simulink library "LopesDevelopmentLibrary"  (R2015b)
settings: Solver=ode45  StartTime=0.0  StopTime=10.0  RelTol=1e-3
values from neighbouring files (symbols this model uses):
  d2r = @(d) d*(pi/180)    [LopesDevelopmentLibrary_LoadParameters.m]
  ts = LopesParams.ts    [LopesDevelopmentLibrary_LoadParameters.m]
undefined symbols (not defined in the file or in its folder): anyParameterChanged, DiscIntNeverNeededParam, gcbh, LHF, LKF, LopesParams, macaddr, mxpcnetworkconfig, mxpcrtudprx, mxpcrtudptx, patientParametersChanged, port, PX, PZ, RHF, RKF, SelectorLOPESInSize, StrideTime_s, Time
undefined symbols (not defined in the file): LopesParamsSendDataArrayLen
libraries: LopesDevelopmentLibrary x288, simulink x98, dspmtrx3 x47, xpciplib x6, xpcnetworkbufferlib x5, dspsigops x4, dspstat3 x3, xpcethernetlib x2, visionstatistics x2, xpcseriallib x2, nmc x1, simulink_extras x1
(part 7 of 12)

== system LopesDevelopmentLibrary/Robot control blocks/ToLopes/GenerateString ==
  note: MaxForces is an array of maximum joint
      | torques and applies to SpringSpring
      | and BiasForceSpring separately.
  UpdateSpringPositions : Inport
  SpringPositions : Inport  Port=2
  SpringVelocities : Inport  Port=3
  SpringStiffnesses : Inport  Port=4
  BiasForces : Inport  Port=5
  MaxForces : Inport  Port=6
  EffectsShouldBeEnabled : Inport  Port=7
  ForceSendEnableEffects : Inport  Port=8
  TreadmillVelocity : Inport  Port=9
  CreateSpringspring : Inport  Port=10
  CreateBiasForceSpring : Inport  Port=11
  Enable : EnablePort
  Detect Change : simulink/Logic and Bit Operations/Detect Change  vinit=0  InputProcessing=Inherited  OutDataTypeStr=boolean
  Detect Change1 : simulink/Logic and Bit Operations/Detect Change  vinit=0  InputProcessing=Inherited  OutDataTypeStr=boolean
  Detect Increase : simulink/Logic and Bit Operations/Detect Increase  vinit=0.0  InputProcessing=Inherited  OutDataTypeStr=boolean
  ForceSendTreadmillVelocity : Constant  Value=false  OutDataTypeStr=boolean
      settings: OpenFcn=|
      | b = get_param(gcb,'value');
      | if (strcmp(b,'true')),
      |   set_param (gcb,'value','false');
      | else
      |   set_param(gcb,'value','true');
      | end;
  Or : Logic  Operator=OR  Inputs=1  AllPortsSameDT=off  OutDataTypeStr=boolean
  OrEnableEffects : Logic  Operator=OR  AllPortsSameDT=off  OutDataTypeStr=boolean
  OrTreadmill : Logic  Operator=OR  AllPortsSameDT=off  OutDataTypeStr=boolean
  ToLopes_GenerateString : S-Function  InitFcn=try, set_param(gcb,'FunctionName','ToLopes_GenerateString'), end  FunctionName=ToLopes_GenerateString  SFunctionModules=ToLopes_GenerateString_wrapper  SFunctionDeploymentMode=off  EnableBusSupport=off  mask(S-Function Builder){}
      mask help: Simulink:masks:SFunctionBuilder_MD
      mask init: same as LopesDevelopmentLibrary/Various/SLRTMessage/S-Function Builder
      settings: CopyFcn=set_param(gcbh,'LinkStatus','none')  PreSaveFcn=try, set_param(gcb,'FunctionName','ToLopes_GenerateString'), end  OpenFcn=sfunctionwizard(gcbh)
      mask Display: plot(val(:,1),val(:,2)),disp(sys), port_label('input',1,'UpdateSpringSpringPositions'), port_label('input',2,'SpringPositions'), port_label('input',3,'SpringVelocities'), port_label('input',4,'SpringStiffnesses'), port_label('input',5,'BiasForces'), port_label('input',6,'MaxForces'), port_label('input',7,'UpdateMaxForces'), port_label('input',8,'TreadmillVelocity'), port_label('input',9,'TreadmillVelocityChanged'), port_label('input',10,'CreateSpringSpring'), port_label('input',11,'CreateBiasForceSpring'), port_label('input',12,'EnableEffects'), port_label('output',1,'s'), port_label('output',2,'s_len')
  s : Outport
  s_len : Outport  Port=2
  wires:
  UpdateSpringPositions/1 -> ToLopes_GenerateString/1
  OrEnableEffects/1 -> ToLopes_GenerateString/12
  Detect Increase/1 -> OrEnableEffects/1
  EffectsShouldBeEnabled/1 -> Detect Increase/1
  ForceSendTreadmillVelocity/1 -> OrTreadmill/2
  OrTreadmill/1 -> ToLopes_GenerateString/9
  Detect Change1/1 -> OrTreadmill/1
  TreadmillVelocity/1 -> ToLopes_GenerateString/8, Detect Change1/1
  SpringVelocities/1 -> ToLopes_GenerateString/3
  Or/1 -> ToLopes_GenerateString/7
  Detect Change/1 -> Or/1
  MaxForces/1 -> ToLopes_GenerateString/6, Detect Change/1
  ForceSendEnableEffects/1 -> OrEnableEffects/2
  CreateSpringspring/1 -> ToLopes_GenerateString/10
  CreateBiasForceSpring/1 -> ToLopes_GenerateString/11
  SpringPositions/1 -> ToLopes_GenerateString/2
  SpringStiffnesses/1 -> ToLopes_GenerateString/4
  ToLopes_GenerateString/2 -> s_len/1
  ToLopes_GenerateString/1 -> s/1
  BiasForces/1 -> ToLopes_GenerateString/5

== system LopesDevelopmentLibrary/Robot control blocks/ToLopes/GenerateVelocities ==
  note: This block allows you to choose different sources for the
      | velocity component of the springspring. Normal behaviour
      | (when ForceVelocityMethod=-1) is that it will use the user-provided
      | velocity if that is an 8-element array, and it will
      | use numerical derivative of the position signal if it the velocity input
      | is a scalar (i.e., in order to use the numerical derivative, you just need to
      | give a scalar constant at the input).
  note: ForceVelocityMethod:
      | -1: Auto (use user-proved velocities if available; use numerical derivative otherwise)
      | 0: ERROR
      | 1: User velocities
      | 2. Numerical Derivatives
      | 3. Filtered numerical derivatives (tau=0.01 s)
      | 4. Zero velocity
  Positions : Inport
  Velocities : Inport  Port=2
  SignalWidth : Inport  Port=3
  ForceVelocityMethod : Inport  Port=4
  Demux : Demux
  MATLAB Function : MATLAB Function  TreatAsAtomicUnit=on
  Merge : Merge  Inputs=4
  UseNumericalDerivative : Subsystem  TreatAsAtomicUnit=on
  UseNumericalDerivativeFiltered : Subsystem  TreatAsAtomicUnit=on
  UseUserVelocity : Subsystem  TreatAsAtomicUnit=on
  UseZeros : Subsystem  TreatAsAtomicUnit=on
  v_out : Outport
  wires:
  Velocities/1 -> UseUserVelocity/1(Velocities_in)
  SignalWidth/1 -> MATLAB Function/1(signalWidth)
  Demux/1 -> UseUserVelocity/Enable
  Positions/1 -> UseNumericalDerivative/1(Positions), UseNumericalDerivativeFiltered/1(Positions)
  Demux/2 -> UseNumericalDerivative/Enable
  ForceVelocityMethod/1 -> MATLAB Function/2(forceType)
  MATLAB Function/1(ena) -> Demux/1
  Demux/4 -> UseZeros/Enable
  Demux/3 -> UseNumericalDerivativeFiltered/Enable
  UseNumericalDerivativeFiltered/1(Velocities) -> Merge/3
  UseZeros/1(Velocities) -> Merge/4
  UseNumericalDerivative/1(Velocities) -> Merge/2
  UseUserVelocity/1(Velocities) -> Merge/1
  Merge/1 -> v_out/1

== system LopesDevelopmentLibrary/Robot control blocks/ToLopes/ParseString ==
  s : Inport
  In2 : Inport  Port=2
  Enable : EnablePort
  ToLopes_ParseString : S-Function  InitFcn=try, set_param(gcb,'FunctionName','ToLopes_ParseString'), end  FunctionName=ToLopes_ParseString  SFunctionModules=ToLopes_ParseString_wrapper  SFunctionDeploymentMode=off  EnableBusSupport=off  mask(S-Function Builder){}
      mask help: Simulink:masks:SFunctionBuilder_MD
      mask init: same as LopesDevelopmentLibrary/Various/SLRTMessage/S-Function Builder
      settings: CopyFcn=set_param(gcbh,'LinkStatus','none')  PreSaveFcn=try, set_param(gcb,'FunctionName','ToLopes_ParseString'), end  OpenFcn=sfunctionwizard(gcbh)
      mask Display: plot(val(:,1),val(:,2)),disp(sys), port_label('input',1,'s'), port_label('input',2,'s_len'), port_label('output',1,'ErrorValue'), port_label('output',2,'SpringSpringDidntExist'), port_label('output',3,'BiasForceSpringDidntExist')
  Error : Outport
  SpringSpringDidntExist : Outport  Port=2
  BiasForceSpringDidntExist : Outport  Port=3
  wires:
  ToLopes_ParseString/3 -> BiasForceSpringDidntExist/1
  ToLopes_ParseString/2 -> SpringSpringDidntExist/1
  ToLopes_ParseString/1 -> Error/1
  s/1 -> ToLopes_ParseString/1
  In2/1 -> ToLopes_ParseString/2

== system LopesDevelopmentLibrary/Robot control blocks/ToLopes/SwitchVelocitiesOnly ==
  note: This block contains the logic for
      | using 'velocity only' control.
      | You should ONLY use it if
      | you have analytical derivatives of your
      | positions. If you have analytical second derivatives
      | as well, it will be more accurate
      | (use the block Various|BetterSpringVelocities)
      |
      | NOTE: UseAnalyticalVelocityOnly is more accurate (i.e., better),
      | but only usable if you have correct derivatives.
  note: The UseAnalyticalVelocityOnly block does not work properly
      | and (thus) should not be used until it's fixed. Please use the positions-and-velocity
      | mode.
      |
      | (the reason this doesn't work: I'm comparing the DesiredSpringPos with the ModelPosIn,
      | but I should compare it to the ActualSpringPos. I don't read that from the LLC yet, and adding
      | this requires some testing. So it is not a 1-minute fix.) - GvO, 151215
  UseAnalVelOnly : Inport
  ModelPosIn : Inport  Port=2
  DesSprPos : Inport  Port=3
  DesSprVel : Inport  Port=4
  Logical Operator : Logic  Operator=NOT  AllPortsSameDT=off  OutDataTypeStr=boolean
  Merge : Merge
  Merge1 : Merge
  Merge2 : Merge
  UseAnalyticalVelocityOnly : Subsystem
  UsePositionsAndVelocities : Subsystem
  UpdateSpringPos : Outport
  SpringPositions : Outport  Port=2
  SpringVelocities : Outport  Port=3
  wires:
  Logical Operator/1 -> UsePositionsAndVelocities/Enable
  UseAnalVelOnly/1 -> UseAnalyticalVelocityOnly/Enable, Logical Operator/1
  DesSprVel/1 -> UsePositionsAndVelocities/2(DesSprVel), UseAnalyticalVelocityOnly/3(DesSprVel)
  DesSprPos/1 -> UsePositionsAndVelocities/1(DesSprPos), UseAnalyticalVelocityOnly/2(DesSprPos)
  ModelPosIn/1 -> UseAnalyticalVelocityOnly/1(ModelPosIn)
  UsePositionsAndVelocities/3(SpringVelocities) -> Merge2/2
  UseAnalyticalVelocityOnly/3(SpringVelocities) -> Merge2/1
  UsePositionsAndVelocities/2(SpringPositions) -> Merge1/2
  UseAnalyticalVelocityOnly/2(SpringPositions) -> Merge1/1
  UsePositionsAndVelocities/1(UpdateSpringPos) -> Merge/2
  UseAnalyticalVelocityOnly/1(UpdateSpringPos) -> Merge/1
  Merge1/1 -> SpringPositions/1
  Merge2/1 -> SpringVelocities/1
  Merge/1 -> UpdateSpringPos/1

== system LopesDevelopmentLibrary/Robot control blocks/ToLopes/~Debug ==

== system LopesDevelopmentLibrary/Robot control blocks/ToLopes/~EnableLogic ==

== system LopesDevelopmentLibrary/Various/GenerateSyncPulseFromPhase/DetectPhaseSignalReset ==
  note: This block detects the event of phase reset (i.e., when it
      | goes from (approximately) 100 to (approximately) 0.
      | It does this by checking whether there is a decrease of at
      | least 50% within one sample time.
  Phase : Inport
  Compare To Constant : simulink/Logic and Bit Operations/Compare To Constant  relop=<  const=-50  OutDataTypeStr=boolean
  Subtract : Sum  Inputs=+-
  Unit Delay : UnitDelay  SampleTime=-1
  PhaseReset : Outport
  wires:
  Phase/1 -> Subtract/1, Unit Delay/1
  Compare To Constant/1 -> PhaseReset/1
  Unit Delay/1 -> Subtract/2
  Subtract/1 -> Compare To Constant/1

== system LopesDevelopmentLibrary/Various/GenerateSyncPulseFromPhase/GenerateRandomValue ==
  note: Generate a uniform random number between Minimum and Maximum each
      | time Trigger rises.
  Maximum : Inport
  Minimum : Inport  Port=2
  Trigger : TriggerPort  PortDimensions=1
  Add : Sum
  Product : Product  RndMeth=Zero
  Subtract : Sum  Inputs=+-
  Uniform Random Number : UniformRandomNumber  Minimum=0  Seed=66
  Out : Outport  InitialOutput=0
  wires:
  Maximum/1 -> Subtract/1
  Uniform Random Number/1 -> Product/1
  Product/1 -> Add/1
  Subtract/1 -> Product/2
  Add/1 -> Out/1
  Minimum/1 -> Add/2, Subtract/2

== system LopesDevelopmentLibrary/BlocksForInternalUse/GaitGeneration/CalculateCartesianPositions/ConvertFromAnkleAnglesToFootAngles ==
  note: Input for s-function,
      | jointAngles:
      | PelvisPosX
      | PelvixPosY
      | PelvisPosZ
      | PelvisAxialAngle
      | PelvisFrontalAngle
      | LHA
      | LHF
      | LHEndorotatoin
      | LKF
      | LAEndorotation
      | LAP
      | LAInversion
      | RHA
      | RHF
      | RHEnorotation
      | RKF
      | RAEndorotation
      | RAP
      | RAInversion
  note: The S-function uses absolute angles for the ankle angle,
      | and I use relative angles (relative to the lower leg).
      | This part converts it. It would be better to use
      | the same thing in both software parts however.
      | (but as long as we don't actuate/measure the ankle
      | angle, it doesn't matter at all.
  In : Inport
  Demux1 : Demux  Outputs=11
  Mux1 : Mux  Inputs=19
  Zero{,1..7} (8 alike) : Constant  Value=0
  Out : Outport
  wires:
  Zero7/1 -> Mux1/19  "RAI"
  Zero6/1 -> Mux1/18  "RAP"
  Zero5/1 -> Mux1/17  "RAE"
  Demux1/8 -> Mux1/16  "RKF"
  Zero4/1 -> Mux1/15  "RHE"
  Demux1/7 -> Mux1/14  "RHF"
  Demux1/6 -> Mux1/13  "RHA"
  Zero3/1 -> Mux1/12  "LAI"
  Zero2/1 -> Mux1/11  "LAP"
  Zero1/1 -> Mux1/10  "LAE"
  Demux1/5 -> Mux1/9  "LKF"
  Zero/1 -> Mux1/8  "LHE"
  Demux1/4 -> Mux1/7  "LHF"
  Demux1/3 -> Mux1/6  "LHA"
  Demux1/11 -> Mux1/5  "POB"
  Demux1/10 -> Mux1/4  "PAX"
  Demux1/9 -> Mux1/2  "PY"
  Demux1/2 -> Mux1/3  "PZ"
  Demux1/1 -> Mux1/1  "PX"
  In/1 -> Demux1/1
  Mux1/1 -> Out/1

== system LopesDevelopmentLibrary/BlocksForInternalUse/GaitGeneration/CalculateCartesianPositions/ExtractPatientParameters ==
  Parameters : Inport
  Bus Selector : BusSelector  OutputSignals=Patient.Mass_kg,Patient.BodyLength_m,Patient.PelvisWidth_m,Patient.PelvisHeight_m,Patient.UpperLegLength_m,Patient.LowerLegLength_m,Patient.FootLength_m,Patient.FootHeight_m,patientParametersChanged
  Data Type Conversion : DataTypeConversion  OutDataTypeStr=double
  Mux : Mux  Inputs=12
  PatientDimensions : Outport
  DimensionsChanged : Outport  Port=2
  wires:
  Data Type Conversion/1 -> DimensionsChanged/1
  Bus Selector/8 -> Mux/11, Mux/12  "<FootHeight_m>"
  Bus Selector/2 -> Mux/2  "<BodyLength_m>"
  Bus Selector/5 -> Mux/6, Mux/5  "<UpperLegLength_m>"
  Bus Selector/3 -> Mux/3  "<PelvisWidth_m>"
  Bus Selector/1 -> Mux/1  "<Mass_kg>"
  Bus Selector/7 -> Mux/9, Mux/10  "<FootLength_m>"
  Bus Selector/9 -> Data Type Conversion/1  "<patientParametersChanged>"
  Mux/1 -> PatientDimensions/1
  Bus Selector/6 -> Mux/7, Mux/8  "<LowerLegLength_m>"
  Parameters/1 -> Bus Selector/1
  Bus Selector/4 -> Mux/4  "<PelvisHeight_m>"

== system LopesDevelopmentLibrary/BlocksForInternalUse/GaitGeneration/CalculateCartesianPositions/OmitAnklesAndToes ==
  In : Inport
  Demux1 : Demux  Outputs=11
  Mux1 : Mux  Inputs=7
  Terminator{,1..3} (4 alike) : Terminator
  Out : Outport
  wires:
  Mux1/1 -> Out/1
  Demux1/10 -> Terminator2/1  "RightHeel"
  Demux1/11 -> Terminator3/1  "RightToe"
  Demux1/6 -> Terminator1/1  "LeftToe"
  Demux1/5 -> Terminator/1  "LeftHeel"
  Demux1/7 -> Mux1/5  "RightHip"
  Demux1/9 -> Mux1/7  "RightAnkle"
  Demux1/1 -> Mux1/1  "Pelvis"
  Demux1/2 -> Mux1/2  "LeftHip"
  Demux1/4 -> Mux1/4  "LeftAnkle"
  Demux1/8 -> Mux1/6  "RightKnee"
  In/1 -> Demux1/1
  Demux1/3 -> Mux1/3  "LeftKnee"

== system LopesDevelopmentLibrary/BlocksForInternalUse/GaitGeneration/CalculateReferenceGait/ActuatedDOFs ==

== system LopesDevelopmentLibrary/BlocksForInternalUse/GaitGeneration/CalculateReferenceGait/CalculateAbductionLeft ==
  note: This version of the CalculateAbduction calculates
      | the derivatives analytically. At the end of the script there is a (commented)
      | Matlab script that calculates the derivatives using the symbolic toolbox. It shows analytically that
      | the velocity is calculated correctly, and the acceleration is too complex to solve for.
      | For the acceleration, I put in random numbers as input and compared the result of my own (optimized) equation
      | and the equation found by Matla Symbolic toolbox. They are equal, so that proves that my equations are all okay.
  note: This block calculates the abduction angle for one leg, given the actual pelvis position and the desired ankle position.
      | It does not take into account rotations of the pelvis, but the deviations from that are so small that that is not a problem.
  Parameters : Inport
  PelvisTZ : Inport  Port=2
  AnkleTZ : Inport  Port=3
  xHF : Inport  Port=4
  xKF : Inport  Port=5
  Bus Selector : BusSelector  OutputSignals=Patient.PelvisWidth_m,Patient.UpperLegLength_m,Patient.LowerLegLength_m
  Demux{,1..3} (4 alike) : Demux  Outputs=3
  MATLAB Function : MATLAB Function  TreatAsAtomicUnit=on
  Signal Conversion : SignalConversion
  isRight : Constant  Value=isRight
  Abduction : Outport
  dAbduction_dx : Outport  Port=2
  d2Abduction_dx2 : Outport  Port=3
  wires:
  isRight/1 -> MATLAB Function/1(isRight)
  PelvisTZ/1 -> Demux/1
  AnkleTZ/1 -> Demux1/1
  xHF/1 -> Demux2/1
  xKF/1 -> Demux3/1
  Parameters/1 -> Bus Selector/1
  Bus Selector/1 -> MATLAB Function/14(w_pelvis)  "<PelvisWidth_m>"
  Bus Selector/2 -> MATLAB Function/15(l_upper)  "<UpperLegLength_m>"
  Bus Selector/3 -> MATLAB Function/16(l_lower)  "<LowerLegLength_m>"
  MATLAB Function/1(Abduction) -> Signal Conversion/1
  MATLAB Function/2(dAbductiondx) -> dAbduction_dx/1
  MATLAB Function/3(ddAbductiondx) -> d2Abduction_dx2/1
  Signal Conversion/1 -> Abduction/1
  Demux/2 -> MATLAB Function/3(dPelvisTZdx)
  Demux/3 -> MATLAB Function/4(ddPelvisTZdx)
  Demux/1 -> MATLAB Function/2(PelvisTZ)
  Demux1/2 -> MATLAB Function/6(dAnkleTZdx)
  Demux1/1 -> MATLAB Function/5(AnkleTZ)
  Demux1/3 -> MATLAB Function/7(ddAnkleTZdx)
  Demux2/2 -> MATLAB Function/9(dxHFdx)
  Demux2/3 -> MATLAB Function/10(ddxHFdx)
  Demux2/1 -> MATLAB Function/8(xHF)
  Demux3/3 -> MATLAB Function/13(ddxKFdx)
  Demux3/1 -> MATLAB Function/11(xKF)
  Demux3/2 -> MATLAB Function/12(dxKFdx)

== system LopesDevelopmentLibrary/BlocksForInternalUse/GaitGeneration/CalculateReferenceGait/CalculateAbductionRight ==
  note: This block calculates the abduction angle for one leg, given the actual pelvis position and the desired ankle position.
      | It does not take into account rotations of the pelvis, but the deviations from that are so small that that is not a problem.
  note: This version of the CalculateAbduction calculates
      | the derivatives analytically. At the end of the script there is a (commented)
      | Matlab script that calculates the derivatives using the symbolic toolbox. It shows analytically that
      | the velocity is calculated correctly, and the acceleration is too complex to solve for.
      | For the acceleration, I put in random numbers as input and compared the result of my own (optimized) equation
      | and the equation found by Matla Symbolic toolbox. They are equal, so that proves that my equations are all okay.
  Parameters : Inport
  PelvisTZ : Inport  Port=2
  AnkleTZ : Inport  Port=3
  xHF : Inport  Port=4
  xKF : Inport  Port=5
  Bus Selector : BusSelector  OutputSignals=Patient.PelvisWidth_m,Patient.UpperLegLength_m,Patient.LowerLegLength_m
  Demux{,1..3} (4 alike) : Demux  Outputs=3
  MATLAB Function : MATLAB Function  TreatAsAtomicUnit=on
  Signal Conversion : SignalConversion
  isRight : Constant  Value=isRight
  Abduction : Outport
  dAbduction_dx : Outport  Port=2
  d2Abduction_dx2 : Outport  Port=3
  wires:
  Demux3/2 -> MATLAB Function/12(dxKFdx)
  Demux3/1 -> MATLAB Function/11(xKF)
  Demux3/3 -> MATLAB Function/13(ddxKFdx)
  Demux2/1 -> MATLAB Function/8(xHF)
  Demux2/3 -> MATLAB Function/10(ddxHFdx)
  Demux2/2 -> MATLAB Function/9(dxHFdx)
  Demux1/3 -> MATLAB Function/7(ddAnkleTZdx)
  Demux1/1 -> MATLAB Function/5(AnkleTZ)
  Demux1/2 -> MATLAB Function/6(dAnkleTZdx)
  Demux/1 -> MATLAB Function/2(PelvisTZ)
  Demux/3 -> MATLAB Function/4(ddPelvisTZdx)
  Demux/2 -> MATLAB Function/3(dPelvisTZdx)
  Signal Conversion/1 -> Abduction/1
  MATLAB Function/3(ddAbductiondx) -> d2Abduction_dx2/1
  MATLAB Function/2(dAbductiondx) -> dAbduction_dx/1
  MATLAB Function/1(Abduction) -> Signal Conversion/1
  Bus Selector/3 -> MATLAB Function/16(l_lower)  "<LowerLegLength_m>"
  Bus Selector/2 -> MATLAB Function/15(l_upper)  "<UpperLegLength_m>"
  Bus Selector/1 -> MATLAB Function/14(w_pelvis)  "<PelvisWidth_m>"
  Parameters/1 -> Bus Selector/1
  xKF/1 -> Demux3/1
  xHF/1 -> Demux2/1
  AnkleTZ/1 -> Demux1/1
  PelvisTZ/1 -> Demux/1
  isRight/1 -> MATLAB Function/1(isRight)

== system LopesDevelopmentLibrary/BlocksForInternalUse/GaitGeneration/CalculateReferenceGait/FirstDerivativeWrtTime ==
  dydx : Inport
  dtdx : Inport  Port=2
  Divide : Product  Inputs=*/
  dydt : Outport
  wires:
  Divide/1 -> dydt/1
  dydx/1 -> Divide/1
  dtdx/1 -> Divide/2

== system LopesDevelopmentLibrary/BlocksForInternalUse/GaitGeneration/CalculateReferenceGait/SecondDerivativeWrtTime ==
  ddydx : Inport
  dtdx : Inport  Port=2
  Divide1 : Product  Inputs=*/
  Math Function : Math  Operator=square  SaturateOnIntegerOverflow=on
  ddydt : Outport
  wires:
  dtdx/1 -> Math Function/1
  Math Function/1 -> Divide1/2
  ddydx/1 -> Divide1/1
  Divide1/1 -> ddydt/1

== system LopesDevelopmentLibrary/BlocksForInternalUse/GaitGeneration/CalculateReferenceGait/Unactuated DOFS ==

== system LopesDevelopmentLibrary/BlocksForInternalUse/GaitGenerationStartStop/ExtraKeyPoints /LeftHipFlexion ==
  parameters : Inport
  SetVelocity : Inport  Port=2
  Bus Creator4 : BusCreator  Inputs=2
  Bus Selector : BusSelector  OutputSignals=General.WalkingVelocity_m_s,Patient.BodyLength_m
  RegressionData : Constant  Value=LopesParams.GaitDataStartLeft.LHF
  RegressionData2KeyEvents : LopesDevelopmentLibrary/BlocksForInternalUse/GaitGeneration/RegressionData2KeyEvents
  Switch : Switch  Criteria=u2 > Threshold
  KeyEvents : Outport
  wires:
  RegressionData2KeyEvents/1 -> KeyEvents/1
  parameters/1 -> Bus Selector/1
  RegressionData/1 -> RegressionData2KeyEvents/1
  Bus Creator4/1 -> RegressionData2KeyEvents/2
  Bus Selector/2 -> Bus Creator4/2  "<BodyLength_m>"
  Bus Selector/1 -> Switch/3  "<WalkingVelocity_m_s>"
  SetVelocity/1 -> Switch/2, Switch/1
  Switch/1 -> Bus Creator4/1  "WalkingVelocity_m_s"

== system LopesDevelopmentLibrary/BlocksForInternalUse/GaitGenerationStartStop/ExtraKeyPoints /LeftKneeFlexion ==
  parameters : Inport
  SetVelocity : Inport  Port=2
  Bus Creator4 : BusCreator  Inputs=2
  Bus Selector : BusSelector  OutputSignals=General.WalkingVelocity_m_s,Patient.BodyLength_m
  RegressionData : Constant  Value=LopesParams.GaitDataStartLeft.LKF
  RegressionData2KeyEvents : LopesDevelopmentLibrary/BlocksForInternalUse/GaitGeneration/RegressionData2KeyEvents
  Switch : Switch  Criteria=u2 > Threshold
  KeyEvents : Outport
  wires:
  RegressionData2KeyEvents/1 -> KeyEvents/1
  RegressionData/1 -> RegressionData2KeyEvents/1
  parameters/1 -> Bus Selector/1
  Bus Creator4/1 -> RegressionData2KeyEvents/2
  Bus Selector/2 -> Bus Creator4/2  "<BodyLength_m>"
  Bus Selector/1 -> Switch/3  "<WalkingVelocity_m_s>"
  SetVelocity/1 -> Switch/2, Switch/1
  Switch/1 -> Bus Creator4/1  "WalkingVelocity_m_s"

== system LopesDevelopmentLibrary/BlocksForInternalUse/GaitGenerationStartStop/ExtraKeyPoints /PelvisTPX ==
  parameters : Inport
  SetVelocity : Inport  Port=2
  Bus Creator4 : BusCreator  Inputs=2
  Bus Selector : BusSelector  OutputSignals=General.WalkingVelocity_m_s,Patient.BodyLength_m
  RegressionData : Constant  Value=LopesParams.GaitDataStartLeft.PX
  RegressionData2KeyEvents : LopesDevelopmentLibrary/BlocksForInternalUse/GaitGeneration/RegressionData2KeyEvents
  Switch : Switch  Criteria=u2 > Threshold
  KeyEvents : Outport
  wires:
  Switch/1 -> Bus Creator4/1  "WalkingVelocity_m_s"
  SetVelocity/1 -> Switch/1, Switch/2
  Bus Selector/1 -> Switch/3  "<WalkingVelocity_m_s>"
  Bus Selector/2 -> Bus Creator4/2  "<BodyLength_m>"
  Bus Creator4/1 -> RegressionData2KeyEvents/2
  RegressionData/1 -> RegressionData2KeyEvents/1
  parameters/1 -> Bus Selector/1
  RegressionData2KeyEvents/1 -> KeyEvents/1

== system LopesDevelopmentLibrary/BlocksForInternalUse/GaitGenerationStartStop/ExtraKeyPoints /PelvisTPZ ==
  parameters : Inport
  SetVelocity : Inport  Port=2
  Bus Creator4 : BusCreator  Inputs=2
  Bus Selector : BusSelector  OutputSignals=General.WalkingVelocity_m_s,Patient.BodyLength_m
  RegressionData : Constant  Value=LopesParams.GaitDataStartLeft.PZ
  RegressionData2KeyEvents : LopesDevelopmentLibrary/BlocksForInternalUse/GaitGeneration/RegressionData2KeyEvents
  Switch : Switch  Criteria=u2 > Threshold
  KeyEvents : Outport
  wires:
  Switch/1 -> Bus Creator4/1  "WalkingVelocity_m_s"
  SetVelocity/1 -> Switch/1, Switch/2
  Bus Selector/1 -> Switch/3  "<WalkingVelocity_m_s>"
  Bus Selector/2 -> Bus Creator4/2  "<BodyLength_m>"
  Bus Creator4/1 -> RegressionData2KeyEvents/2
  RegressionData/1 -> RegressionData2KeyEvents/1
  parameters/1 -> Bus Selector/1
  RegressionData2KeyEvents/1 -> KeyEvents/1

== system LopesDevelopmentLibrary/BlocksForInternalUse/GaitGenerationStartStop/ExtraKeyPoints /RightHipFlexion ==
  parameters : Inport
  SetVelocity : Inport  Port=2
  Bus Creator4 : BusCreator  Inputs=2
  Bus Selector : BusSelector  OutputSignals=General.WalkingVelocity_m_s,Patient.BodyLength_m
  RegressionData : Constant  Value=LopesParams.GaitDataStartLeft.RHF
  RegressionData2KeyEvents : LopesDevelopmentLibrary/BlocksForInternalUse/GaitGeneration/RegressionData2KeyEvents
  Switch : Switch  Criteria=u2 > Threshold
  KeyEvents : Outport
  wires:
  RegressionData/1 -> RegressionData2KeyEvents/1
  RegressionData2KeyEvents/1 -> KeyEvents/1
  parameters/1 -> Bus Selector/1
  Bus Creator4/1 -> RegressionData2KeyEvents/2
  Bus Selector/2 -> Bus Creator4/2  "<BodyLength_m>"
  Bus Selector/1 -> Switch/3  "<WalkingVelocity_m_s>"
  SetVelocity/1 -> Switch/2, Switch/1
  Switch/1 -> Bus Creator4/1  "WalkingVelocity_m_s"

== system LopesDevelopmentLibrary/BlocksForInternalUse/GaitGenerationStartStop/ExtraKeyPoints /RightKneeFlexion ==
  parameters : Inport
  SetVelocity : Inport  Port=2
  Bus Creator4 : BusCreator  Inputs=2
  Bus Selector : BusSelector  OutputSignals=General.WalkingVelocity_m_s,Patient.BodyLength_m
  RegressionData : Constant  Value=LopesParams.GaitDataStartLeft.RKF
  RegressionData2KeyEvents : LopesDevelopmentLibrary/BlocksForInternalUse/GaitGeneration/RegressionData2KeyEvents
  Switch : Switch  Criteria=u2 > Threshold
  KeyEvents : Outport
  wires:
  RegressionData2KeyEvents/1 -> KeyEvents/1
  RegressionData/1 -> RegressionData2KeyEvents/1
  parameters/1 -> Bus Selector/1
  Bus Creator4/1 -> RegressionData2KeyEvents/2
  Bus Selector/2 -> Bus Creator4/2  "<BodyLength_m>"
  Bus Selector/1 -> Switch/3  "<WalkingVelocity_m_s>"
  SetVelocity/1 -> Switch/2, Switch/1
  Switch/1 -> Bus Creator4/1  "WalkingVelocity_m_s"

== system LopesDevelopmentLibrary/BlocksForInternalUse/GaitGenerationStartStop/ExtraKeyPoints /TimeCalculation ==
  StrideTime : Inport
  Bus Creator7 : BusCreator  Inputs=2
  Constant : Constant  Value=[0,0,1; 100,1,1]
  Gain : Gain  Gain=0.01
  Mux : Mux  Inputs=2
  Overwrite Values : dspmtrx3/Overwrite Values  OverWriteDiag=Submatrix  valFrom2ndIP=Second input port  ConstValue=0  RowSpan=One row  RowStartMode=Index  RowStartIndex=2  RowEndMode=Last  RowEndIndex=1  ColSpan=One column  ColStartMode=Index  ColStartIndex=2  ColEndMode=Last  ColEndIndex=1  DiagSpan=Range of elements  DiagStartMode=Index  DiagStartIndex=2  DiagEndMode=Index  DiagEndIndex=4
  Overwrite Values1 : dspmtrx3/Overwrite Values  OverWriteDiag=Submatrix  valFrom2ndIP=Second input port  ConstValue=0  RowSpan=All rows  RowStartMode=Index  RowStartIndex=2  RowEndMode=Last  RowEndIndex=1  ColSpan=One column  ColStartMode=Last  ColStartIndex=2  ColEndMode=Last  ColEndIndex=1  DiagSpan=Range of elements  DiagStartMode=Index  DiagStartIndex=2  DiagEndMode=Index  DiagEndIndex=4
  Time : LopesDevelopmentLibrary/BlocksForInternalUse/GaitGeneration/keyEvents2breakscoefs3  SystemSampleTime=-1
  BreaksCoefsTime : Outport
  wires:
  StrideTime/1 -> Overwrite Values/2, Gain/1
  Overwrite Values1/1 -> Time/1
  Constant/1 -> Overwrite Values/1
  Overwrite Values/1 -> Overwrite Values1/1
  Mux/1 -> Overwrite Values1/2
  Gain/1 -> Mux/1, Mux/2  "slope"
  Time/2 -> Bus Creator7/2
  Time/1 -> Bus Creator7/1
  Bus Creator7/1 -> BreaksCoefsTime/1  "Time"

== system LopesDevelopmentLibrary/BlocksForInternalUse/LLC Communication/LLC Network Configuration/Variant Network Init ==
  note: 1) Only subsystems can be added as variant choices at this level
      | 2) Blocks cannot be connected at this level as connectivity is
      | automatically determined at simulation, based on the active variant
  note: I did not remove the inputs/outputs because that makes Matlab fail...
  Dummy_in : Inport
  Init_NonRT_UDP : Subsystem  VariantControl=LopesVariant_Non_RT
  Init_RT_2012b : Subsystem  VariantControl=LopesVariant_RT_2012b
  Init_RT_2014b : Subsystem  VariantControl=LopesVariant_RT_2014b
  Init_RT_2015b : Subsystem  VariantControl=LopesVariant_RT_2015b
  Dummy_out : Outport

== system LopesDevelopmentLibrary/BlocksForInternalUse/LLC Communication/LLCReceiveUDP/Debug ==

== system LopesDevelopmentLibrary/BlocksForInternalUse/LLC Communication/LLCReceiveUDP/UDPReceiveVariantChannel ==
  note: 1) Add Subsystem or Model blocks as valid variant choices.
      | 2) You cannot connect blocks at this level. At simulation, connectivity is automatically
      | determined, based on the active variant and port name matching.
  Dummy_in : Inport
  Receive_Non_RT : Subsystem  VariantControl=LopesVariant_Non_RT
  Receive_RT_2015b : Subsystem  VariantControl=LopesVariant_RT_2015b
  Receive_RT_R2012b : Subsystem  VariantControl=LopesVariant_RT_2012b
  Receive_RT_R2014b : Subsystem  VariantControl=LopesVariant_RT_2014b
  RecvData : Outport
  RecvLen : Outport  Port=2

== system LopesDevelopmentLibrary/BlocksForInternalUse/LLC Communication/LLCSendUDP/Debug ==

== system LopesDevelopmentLibrary/BlocksForInternalUse/LLC Communication/LLCSendUDP/UDPSendVariant ==
  Data : Inport
  Len : Inport  Port=2
  Enable : EnablePort
  Terminator : Terminator
  UDPSendVariantChannel : Subsystem  Variant=on
  wires:
  Data/1 -> UDPSendVariantChannel/1(SendData)
  Len/1 -> UDPSendVariantChannel/2(SendLen)
  UDPSendVariantChannel/1(Dummy_out) -> Terminator/1

== system LopesDevelopmentLibrary/BlocksForInternalUse/LLC Communication/UDP_Blocks/Network Configuration_RT_2012b  ==
  "ARP Init " : S-Function  Priority=0  FunctionName=xpcdebugarpinit  Parameters=Stats, Interface, IpAddress, SubnetMask, Gateway, EthernetId, Flags, BlockId, Retry, Timeout, Expiration, StaticAddressListIp, StaticAddressListMac, DiscoveryList, MulticastList, SampleTime  SFunctionDeploymentMode=off  EnableBusSupport=off  mask(arpinit){Interface=0, IpAddress=IpAddress, SubnetMask=SubnetMask, Gateway=Gateway, EthernetId=1, BlockId=0, SampleTime=-1, Flags=hex2dec('00000697'), Stats=off, Retry=5, Timeout=20, Expiration=20*60, StaticAddressListIp=[], StaticAddressListMac=[], DiscoveryList=[], MulticastList=[]}
      mask prompts: IpAddress "IP Address"; SubnetMask "Subnet Mask"; EthernetId "Ethernet ID"; BlockId "Block ID"; SampleTime "Sample Time"; Stats "Statistics Port"; StaticAddressListIp "[Static IP]"; StaticAddressListMac "[Static MAC]"; DiscoveryList "[Discovery IP]"; MulticastList "[Multicast IP]"
      mask help: ARP Init
      mask init:
      | xpclinklib('xpciplib');
      mask Help: web('arpdebug.htm',  '-helpbrowser');
      mask Display: disp('ARP Init');
  "Buffer Mngmt " : S-Function  Priority=-1  FunctionName=xpcnb  Parameters=pool_sizes, SampleTime, ShowTune  SFunctionDeploymentMode=off  EnableBusSupport=off  mask(xpcnbinit){SampleTime=-1, PoolSizes=[100 10 10 200], ShowTune=off}
      mask prompts: SampleTime "Sample time:"; PoolSizes "Buffer pool sizes (256, 512, 1024, 2048):"; ShowTune "Display tuning information"
      mask help: Network Buffer Initialization
      mask init:
      | [MaskDisplay, pool_sizes] = mxpcnbinit(2, PoolSizes);
      | 
      | set_param(gcb, 'MaskDisplay', MaskDisplay);
      mask Help: eval('xpcdoc(''NB_Init'')');
      mask Display: disp('Network Buffer\nManagement');
  "Ethernet Init " : S-Function  Priority=-1  FunctionName=xpcetherinit  Parameters="ID, Driver, Bus, Slot, VendorID, DeviceID, AddressSource, mac, TxSA, RxPromiscuous, RxBad, RxShort, MaxMTU, TxThreshold, TxBuffers, RxBuffers, ShowTune, numMulti, multicast,   NumRxBlks, SampleTime"  SFunctionDeploymentMode=off  EnableBusSupport=off  mask(xpcetherinit){ID=1, Driver=EthDrv, Bus=PciBus, Slot=PciSlot, SampleTime=-1, AddressSource=EEPROM, MAC=macaddr('00:00:00:00:00:00'), TxSA=off, RxPromiscuous=off, Multicast={}, RxBad=off, RxShort=off, MaxMTU=1518, TxThreshold=224, TxBuffers=128, RxBuffers=64, ShowTune=off, NumRxBlks=1}
      mask prompts: ID "Device ID:"; Bus "PCI bus:"; Slot "PCI slot:"; SampleTime "Sample time:"; AddressSource "Address source:"; TxSA "Tx source address from model"; RxPromiscuous "Rx promiscuous"; Multicast "Multicast address list:"; RxBad "Rx bad frames"; RxShort "Rx short frames"; MaxMTU "Max MTU:"; TxThreshold "Tx threshold:"; TxBuffers "Tx buffers:"; RxBuffers "Rx buffers:"; ShowTune "Display tuning information"; NumRxBlks "num rx blocks"
      mask help: Ethernet Initialization
      mask init:
      | VendorID = -1;
      | DeviceID = -1;
      | 
      | [MaskDisplay, VendorID, DeviceID, mac, numMulti, multicast] = mxpcetherinit(2, ID, Driver, Bus, Slot, MAC, Multicast);
      | 
      | set_param(gcb, 'MaskDisplay', MaskDisplay);
      mask Help: eval('xpcdoc(''Ether_Init'')');
      mask TypeOptions ID: 1 | 2 | 3 | 4 | 5 | 6 | 7 | 8
      mask TypeOptions AddressSource: EEPROM | Specify
      mask Callback AddressSource:
      | enables = get_param(gcb, 'MaskVisibilities');
      | if strcmp('Specify', get_param(gcb, 'AddressSource'))
      |     enables{strmatch('MAC',fieldnames(get_param(gcb,'DialogParameters')))} = 'on';
      | else
      |     enables{strmatch('MAC',fieldnames(get_param(gcb,'DialogParameters')))} = 'off';
      | end
      | set_param(gcb, 'MaskVisibilities', enables);
      mask Display: disp('Ethernet\nInitialization\nbus: 1 slot: 0\nId: 1\nIntel Gigabit');
  "IP Init " : S-Function  Priority=1  FunctionName=xpcdebugipinit  Parameters=Stats, Group, ArpId, IpAddress, SubnetMask, DefaultGateway, DefaultInterface, Flags, ToS, StartingId, TTL, SampleTime  SFunctionDeploymentMode=off  EnableBusSupport=off  mask(ipinit){Group=0, ArpId=[0], IpAddress=[IpAddress], SubnetMask=[SubnetMask], DefaultGateway=Gateway, DefaultInterface=0, SampleTime=-1, Flags=hex2dec('00000005'), ToS=hex2dec('00'), StartingId=10000, TTL=64, Stats=off}
      mask prompts: ArpId "[ARP ID]"; IpAddress "[IP Address]"; SubnetMask "[Subnet Mask]"; DefaultGateway "Default Gateway"; DefaultInterface "Default Interface"; SampleTime "Sample Time"; StartingId "Starting Id"; Stats "Statistics Port"
      mask help: IP Init
      mask init:
      | xpclinklib('xpciplib');
      mask Help: web('ipdebug.htm',  '-helpbrowser');
      mask Display: disp('IP Init');
  "UDP Init " : S-Function  Priority=2  FunctionName=xpcdebugudpinit  Parameters=Stats, Group, StartingPort, Flags, SampleTime  SFunctionDeploymentMode=off  EnableBusSupport=off  mask(udpinit){Group=0, StartingPort=10000, Flags=hex2dec('00000001'), SampleTime=-1, Stats=off}
      mask prompts: StartingPort "Starting Port"; SampleTime "Sample Time"; Stats "Statistics Port"
      mask help: UDP Init
      mask init:
      | xpclinklib('xpciplib');
      mask Help: web('udpdebug.htm',  '-helpbrowser');
      mask Display: disp('UDP Init');

== system LopesDevelopmentLibrary/BlocksForInternalUse/LLC Communication/UDP_Blocks/Network Configuration_RT_2014b  ==
  "ARP Init " : S-Function  Priority=0  FunctionName=xpcdebugarpinit  Parameters=Stats, Interface, IpAddress, SubnetMask, Gateway, EthernetId, Flags, BlockId, Retry, Timeout, Expiration, StaticAddressListIp, StaticAddressListMac, DiscoveryList, MulticastList, SampleTime  SFunctionDeploymentMode=off  EnableBusSupport=off  mask(arpinit){Interface=udpID, IpAddress=IpAddress, SubnetMask=SubnetMask, Gateway=Gateway, EthernetId=ID, BlockId=0, SampleTime=-1, Flags=hex2dec('00000697'), Stats=off, Retry=5, Timeout=20, Expiration=20*60, StaticAddressListIp=[], StaticAddressListMac=[], DiscoveryList=[], MulticastList=[]}
      mask prompts: IpAddress "IP Address"; SubnetMask "Subnet Mask"; EthernetId "Ethernet ID"; BlockId "Block ID"; SampleTime "Sample Time"; Stats "Statistics Port"; StaticAddressListIp "[Static IP]"; StaticAddressListMac "[Static MAC]"; DiscoveryList "[Discovery IP]"; MulticastList "[Multicast IP]"
      mask help: ARP Init
      mask init:
      | xpclinklib('xpciplib');
      mask Help: web('arpdebug.htm',  '-helpbrowser');
      mask Display: disp('ARP Init');
  "Buffer Mngmt " : xpcnetworkbufferlib/Buffer Mngmt   Priority=-1  SampleTime=-1  PoolSizes=[100 10 10 200]  ShowTune=off
  "Ethernet Init " : xpcethernetlib/Ethernet Init   Priority=-1  ID=1  Driver=Intel Gigabit  Bus=PciBus  Slot=PciSlot  SampleTime=-1  AddressSource=EEPROM  MAC=macaddr('00:00:00:00:00:00')  TxSA=off  RxPromiscuous=off  Multicast={}  RxBad=off  RxShort=off  MaxMTU=1518  TxThreshold=224  TxBuffers=128  RxBuffers=64  ShowTune=off  NumRxBlks=1
  "IP Init " : S-Function  Priority=1  FunctionName=xpcdebugipinit  Parameters=Stats, Group, ArpId, IpAddress, SubnetMask, DefaultGateway, DefaultInterface, Flags, ToS, StartingId, TTL, SampleTime  SFunctionDeploymentMode=off  EnableBusSupport=off  mask(ipinit){Group=udpID, ArpId=[udpID], IpAddress=[IpAddress], SubnetMask=[SubnetMask], DefaultGateway=Gateway, DefaultInterface=0, SampleTime=-1, Flags=hex2dec('00000005'), ToS=hex2dec('00'), StartingId=10000, TTL=64, Stats=off}
      mask prompts: ArpId "[ARP ID]"; IpAddress "[IP Address]"; SubnetMask "[Subnet Mask]"; DefaultGateway "Default Gateway"; DefaultInterface "Default Interface"; SampleTime "Sample Time"; StartingId "Starting Id"; Stats "Statistics Port"
      mask help: IP Init
      mask init:
      | xpclinklib('xpciplib');
      mask Help: web('ipdebug.htm',  '-helpbrowser');
      mask Display: disp('IP Init');
  "UDP Init " : S-Function  Priority=2  FunctionName=xpcdebugudpinit  Parameters=Stats, Group, StartingPort, Flags, SampleTime  SFunctionDeploymentMode=off  EnableBusSupport=off  mask(udpinit){Group=udpID, StartingPort=10000, Flags=hex2dec('00000001'), SampleTime=-1, Stats=off}
      mask prompts: StartingPort "Starting Port"; SampleTime "Sample Time"; Stats "Statistics Port"
      mask help: UDP Init
      mask init:
      | xpclinklib('xpciplib');
      mask Help: web('udpdebug.htm',  '-helpbrowser');
      mask Display: disp('UDP Init');

== system LopesDevelopmentLibrary/BlocksForInternalUse/LLC Communication/UDP_Blocks/Network Configuration_RT_2015b ==
  "ARP Init " : S-Function  Priority=0  FunctionName=xpcdebugarpinit  Parameters=Stats, Interface, IpAddress, SubnetMask, Gateway, EthernetId, Flags, BlockId, Retry, Timeout, Expiration, StaticAddressListIp, StaticAddressListMac, DiscoveryList, MulticastList, SampleTime  SFunctionDeploymentMode=off  EnableBusSupport=off  mask(arpinit){Interface=udpID, IpAddress=IpAddress, SubnetMask=SubnetMask, Gateway=Gateway, EthernetId=ID, BlockId=0, SampleTime=-1, Flags=hex2dec('00000697'), Stats=off, Retry=5, Timeout=20, Expiration=20*60, StaticAddressListIp=[], StaticAddressListMac=[], DiscoveryList=[], MulticastList=MulticastList}
      mask prompts: IpAddress "IP Address"; SubnetMask "Subnet Mask"; EthernetId "Ethernet ID"; BlockId "Block ID"; SampleTime "Sample Time"; Stats "Statistics Port"; StaticAddressListIp "[Static IP]"; StaticAddressListMac "[Static MAC]"; DiscoveryList "[Discovery IP]"; MulticastList "[Multicast IP]"
      mask help: ARP Init
      mask init:
      | xpclinklib('xpciplib');
      mask Help: web('arpdebug.htm',  '-helpbrowser');
      mask Display: disp('ARP Init');
  "Buffer Mngmt " : xpcnetworkbufferlib/Buffer Mngmt   Priority=-1  SampleTime=-1  PoolSizes=[100 10 10 200]  ShowTune=off
  "Ethernet Init " : xpcethernetlib/Ethernet Init   Priority=-1  ID=1  Driver=Intel Gigabit  Bus=PciBus  Slot=PciSlot  SampleTime=-1  AddressSource=EEPROM  MAC=macaddr('00:00:00:00:00:00')  TxSA=off  RxPromiscuous=off  Multicast=Multicast  RxBad=off  RxShort=off  MaxMTU=1518  TxThreshold=224  TxBuffers=128  RxBuffers=64  ShowTune=off  NumRxBlks=1
  "IP Init " : S-Function  Priority=1  FunctionName=xpcdebugipinit  Parameters=Stats, Group, ArpId, IpAddress, SubnetMask, DefaultGateway, DefaultInterface, Flags, ToS, StartingId, TTL, SampleTime  SFunctionDeploymentMode=off  EnableBusSupport=off  mask(ipinit){Group=udpID, ArpId=[udpID], IpAddress=[IpAddress], SubnetMask=[SubnetMask], DefaultGateway=Gateway, DefaultInterface=0, SampleTime=-1, Flags=hex2dec('00000005'), ToS=hex2dec('00'), StartingId=10000, TTL=64, Stats=off}
      mask prompts: ArpId "[ARP ID]"; IpAddress "[IP Address]"; SubnetMask "[Subnet Mask]"; DefaultGateway "Default Gateway"; DefaultInterface "Default Interface"; SampleTime "Sample Time"; StartingId "Starting Id"; Stats "Statistics Port"
      mask help: IP Init
      mask init:
      | xpclinklib('xpciplib');
      mask Help: web('ipdebug.htm',  '-helpbrowser');
      mask Display: disp('IP Init');
  "UDP Init " : S-Function  Priority=2  FunctionName=xpcdebugudpinit  Parameters=Stats, Group, StartingPort, Flags, SampleTime  SFunctionDeploymentMode=off  EnableBusSupport=off  mask(udpinit){Group=udpID, StartingPort=10000, Flags=hex2dec('00000001'), SampleTime=-1, Stats=off}
      mask prompts: StartingPort "Starting Port"; SampleTime "Sample Time"; Stats "Statistics Port"
      mask help: UDP Init
      mask init:
      | xpclinklib('xpciplib');
      mask Help: web('udpdebug.htm',  '-helpbrowser');
      mask Display: disp('UDP Init');

== system LopesDevelopmentLibrary/BlocksForInternalUse/LLC Communication/UDP_Blocks/Receive_RT_2012b  ==
  "Buffer " : S-Function  FunctionName=xpcnbbuffer  Parameters=chainSize, bufferSize, Threshold  SFunctionDeploymentMode=off  EnableBusSupport=off  mask(xpcnbbuffer){ChainSize=1, BufferSize=0, Threshold=0}
      mask prompts: ChainSize "Chain size:"; BufferSize "Buffer size:"
      mask help:
      | Network Buffer Buffering
      |
      | Chain size = inf --> No buffering, all packets passed through
      | Chain size = 0   --> Deletes all packets, none passed through
      | Chain size > 0   --> Passes through first "Chain size" packets
      | Chain size < 0   --> Passes through last "Chain size" packets
      |
      | Buffer size = inf --> All remaining packets are buffered, none are deleted
      | Buffer size = 0   --> No buffering, deletes all remaining packets
      | Buffer size > 0   --> Buffers remaining first "Buffer size" packets
      | Buffer size < 0   --> Buffers remaining last "Buffer size" packets
      |
      | Threshold = 0 --> No threshold
      | Threshold > 0 --> Delay passing through packets till threshold is met once
      | Threshold < 0 --> Passes through packets if "Threshold" packets are buffered
      mask init:
      | [MaskDisplay, chainSize, bufferSize] = mxpcnbbuffer(2, ChainSize, BufferSize, Threshold);
      | 
      | set_param(gcb, 'MaskDisplay', MaskDisplay);
      mask Help: helpview(fullfile(docroot, 'mapfiles', 'xpc.map'), 'NB_Buffer')
      mask Display: disp('NB\nBuffering\n\n');port_label('output', 1, '1');
  "Extract " : S-Function  FunctionName=xpcnbextract  Parameters=packetSize  SFunctionDeploymentMode=off  EnableBusSupport=off  mask(xpcnbextract){PacketSize=Receive3}
      mask prompts: PacketSize "Packet size (-1: inherit):"
      mask help: Network Buffer Extract
      mask init:
      | [packetSize] = mxpcnbextract(2,PacketSize);
      mask Help: helpview(fullfile(docroot, 'mapfiles', 'xpc.map'), 'NB_Extract')
      mask Display: disp('NB Extract\n');port_label('output', 2, 'length');
  Terminator : Terminator
  "UDP Consume " : S-Function  FunctionName=xpcudpconsume  Parameters=Group, VectorSize, SampleTime  SFunctionDeploymentMode=off  EnableBusSupport=off  mask(udpconsume){Group=0, VectorSize=0, SampleTime=Receive4}
      mask prompts: Group "IP Group"; VectorSize "Output port width:"; SampleTime "Sample time:"
      mask help: UDP Consume
      mask Help: helpview(fullfile(docroot, 'mapfiles', 'xpc.map'), 'RT_UDP_CONSUME')
      mask Display:
      | if VectorSize
      |     disp('UDP Consume\n\n\n\n\n\n\n');
      |     port_label('output', 1, 'Buffers');
      |     port_label('output', 2, 'Source IP Address');
      |     port_label('output', 3, 'Destination IP Address');
      |     port_label('output', 4, 'Local UDP Port');
      |     port_label('output', 5, 'Remote UDP Port');
      |     port_label('output', 6, 'Chain Size');
      | else
      |     disp('UDP Consume');
      |     port_label('output', 1, 'Buffers');
      |     port_label('output', 2, 'Chain Size');
      | end
  "UDP Rx " : S-Function  Priority=5  FunctionName=xpcudprx  Parameters=Group, SourceAddress, sip, LocalPort, lup, SampleTime  SFunctionDeploymentMode=off  EnableBusSupport=off  mask(udprx){Group=0, sip=Any, SourceAddress=Receive1, lup=Specify, LocalPort=Receive2, SampleTime=Receive4}
      mask prompts: Group "IP Group"; sip "Source IP Address"; SourceAddress "IP address to receive from (0.0.0.0 for accepting all):"; lup "Local UDP Port"; LocalPort "IP port to receive from:"; SampleTime "Sample time:"
      mask help: UDP Rx
      mask init:
      | if SourceAddress == 0
      |     sip = 3;
      | end
      | 
      | SourceAddress = ipaddr(SourceAddress);
      mask Help: helpview(fullfile(docroot, 'mapfiles', 'xpc.map'), 'RT_UDP_RX')
      mask TypeOptions sip: Specify | Port | Any
      mask TypeOptions lup: Specify | Port | Any
      mask Display: disp('UDP Rx');
  Out1 : Outport  OutDataTypeStr=uint8
  Out2 : Outport  Port=2  OutDataTypeStr=double
  wires:
  "UDP Consume "/2 -> Terminator/1
  "UDP Consume "/1 -> "Extract "/1
  "UDP Rx "/1 -> "Buffer "/1
  "Buffer "/1 -> "UDP Consume "/1
  "Extract "/1 -> Out1/1
  "Extract "/2 -> Out2/1

== system LopesDevelopmentLibrary/BlocksForInternalUse/LLC Communication/UDP_Blocks/Receive_RT_2014b  ==
  "Buffer " : S-Function  FunctionName=xpcnbbuffer  Parameters=chainSize, bufferSize, Threshold  SFunctionDeploymentMode=off  EnableBusSupport=off  mask(xpcnbbuffer){ChainSize=1, BufferSize=0, Threshold=0}
      mask prompts: ChainSize "Chain size:"; BufferSize "Buffer size:"
      mask help:
      | Network Buffer Buffering
      |
      | Chain size = inf --> No buffering, all packets passed through
      | Chain size = 0   --> Deletes all packets, none passed through
      | Chain size > 0   --> Passes through first "Chain size" packets
      | Chain size < 0   --> Passes through last "Chain size" packets
      |
      | Buffer size = inf --> All remaining packets are buffered, none are deleted
      | Buffer size = 0   --> No buffering, deletes all remaining packets
      | Buffer size > 0   --> Buffers remaining first "Buffer size" packets
      | Buffer size < 0   --> Buffers remaining last "Buffer size" packets
      |
      | Threshold = 0 --> No threshold
      | Threshold > 0 --> Delay passing through packets till threshold is met once
      | Threshold < 0 --> Passes through packets if "Threshold" packets are buffered
      mask init:
      | [MaskDisplay, chainSize, bufferSize] = mxpcnbbuffer(2, ChainSize, BufferSize, Threshold);
      | 
      | set_param(gcb, 'MaskDisplay', MaskDisplay);
      mask Help: helpview(fullfile(docroot, 'mapfiles', 'xpc.map'), 'NB_Buffer')
      mask Display: disp('NB\nBuffering\n\n');port_label('output', 1, '1');
  "Extract " : S-Function  FunctionName=xpcnbextract  Parameters=packetSize  SFunctionDeploymentMode=off  EnableBusSupport=off  mask(xpcnbextract){PacketSize=Receive3}
      mask prompts: PacketSize "Packet size (-1: inherit):"
      mask help: Network Buffer Extract
      mask init:
      | [packetSize] = mxpcnbextract(2,PacketSize);
      mask Help: helpview(fullfile(docroot, 'mapfiles', 'xpc.map'), 'NB_Extract')
      mask Display: disp('NB Extract\n');port_label('output', 2, 'length');
  Terminator : Terminator
  "UDP Consume " : S-Function  FunctionName=xpcudpconsume  Parameters=Group, VectorSize, SampleTime  SFunctionDeploymentMode=off  EnableBusSupport=off  mask(udpconsume){Group=udpID, VectorSize=0, SampleTime=Receive4}
      mask prompts: Group "IP Group"; VectorSize "Output port width:"; SampleTime "Sample time:"
      mask help: UDP Consume
      mask Help: helpview(fullfile(docroot, 'mapfiles', 'xpc.map'), 'RT_UDP_CONSUME')
      mask Display:
      | if VectorSize
      |     disp('UDP Consume\n\n\n\n\n\n\n');
      |     port_label('output', 1, 'Buffers');
      |     port_label('output', 2, 'Source IP Address');
      |     port_label('output', 3, 'Destination IP Address');
      |     port_label('output', 4, 'Local UDP Port');
      |     port_label('output', 5, 'Remote UDP Port');
      |     port_label('output', 6, 'Chain Size');
      | else
      |     disp('UDP Consume');
      |     port_label('output', 1, 'Buffers');
      |     port_label('output', 2, 'Chain Size');
      | end
  "UDP Rx " : S-Function  Priority=5  FunctionName=xpcudprx  Parameters=Group, SourceAddress, sip, LocalPort, lup, SampleTime  SFunctionDeploymentMode=off  EnableBusSupport=off  mask(udprx){Group=udpID, sip=Any, SourceAddress=Receive1, lup=Specify, LocalPort=Receive2, SampleTime=Receive4}
      mask prompts: Group "IP Group"; sip "Source IP Address"; SourceAddress "IP address to receive from (0.0.0.0 for accepting all):"; lup "Local UDP Port"; LocalPort "IP port to receive from:"; SampleTime "Sample time:"
      mask help: UDP Rx
      mask init:
      | if SourceAddress == 0
      |     sip = 3;
      | else
      |     sip = 1;
      | end
      mask Help: helpview(fullfile(docroot, 'mapfiles', 'xpc.map'), 'RT_UDP_RX')
      mask TypeOptions sip: Specify | Port | Any
      mask TypeOptions lup: Specify | Port | Any
      mask Display: disp('UDP Rx');
  Out1 : Outport  OutDataTypeStr=uint8
  Out2 : Outport  Port=2  OutDataTypeStr=double
  wires:
  "UDP Consume "/2 -> Terminator/1
  "UDP Consume "/1 -> "Extract "/1
  "UDP Rx "/1 -> "Buffer "/1
  "Buffer "/1 -> "UDP Consume "/1
  "Extract "/1 -> Out1/1
  "Extract "/2 -> Out2/1
